simulink model "Dinamic_3_day_data_General"  (R2014b)
settings: Solver=ode45  StartTime=0.0  StopTime=255600  FixedStep=3600  RelTol=1e-3
undefined symbols (not defined in the file or in its folder): date_3, Dry_bulb_3, GHI_3
libraries: simulink x1
settings Model: Creator=Timur  LastModifiedBy=Timur
settings SolverCC: InitialStep=1000  ZeroCrossAlgorithm=Adaptive
settings DebuggingCC: AlgebraicLoopMsg=none  MaxConsecutiveZCsMsg=none  SolverPrmCheckMsg=none

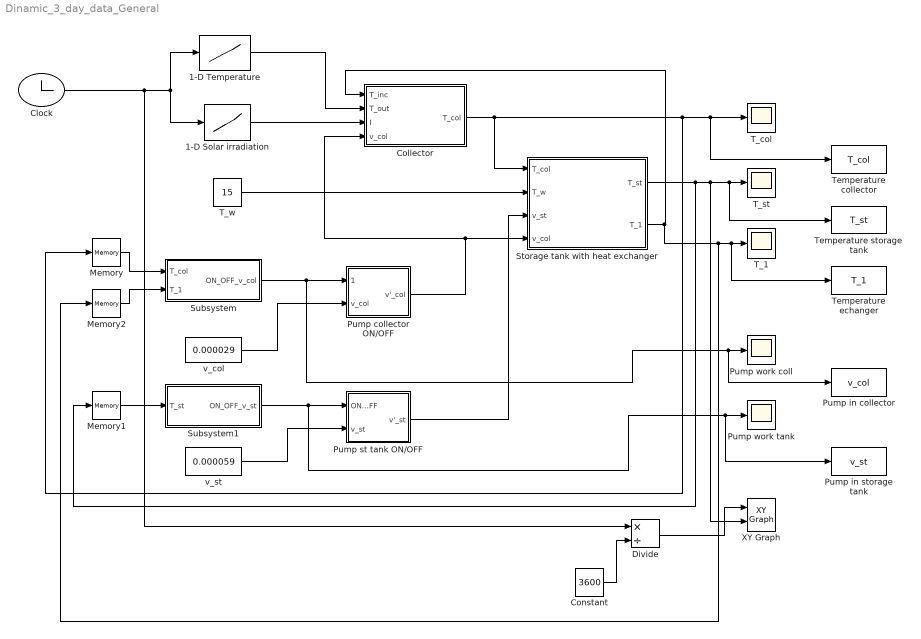
== system Dinamic_3_day_data_General ==
  1-D Solar irradiation : Lookup_n-D  NumberOfTableDimensions=1  BreakpointsForDimension1=date_3  Table=GHI_3  InterpMethod=Cubic spline  SampleTime=3600  InternalRulePriority=Speed  RndMeth=Simplest  InputSameDT=on
  1-D Temperature : Lookup_n-D  NumberOfTableDimensions=1  BreakpointsForDimension1=date_3  Table=Dry_bulb_3  InterpMethod=Cubic spline  SampleTime=3600  InternalRulePriority=Speed  RndMeth=Simplest  InputSameDT=on
  Clock : Clock
  Collector : Subsystem
  Constant : Constant  Value=3600
  Divide : Product  Inputs=*/
  Memory : Memory
  Memory1 : Memory
  Memory2 : Memory
  Pump collector ON/OFF : Subsystem
  Pump in collector : ToWorkspace  VariableName=v_col  SaveFormat=Timeseries  SampleTime=-1
  Pump in storage tank : ToWorkspace  VariableName=v_st  SaveFormat=Timeseries  SampleTime=-1
  Pump st tank ON/OFF : Subsystem
  Pump work coll : Scope
      settings: YMin=0  YMax=1  SaveName=ScopeData3
  Pump work tank : Scope
      settings: YMin=-1  YMax=1  SaveName=ScopeData4
  Storage tank with heat exchanger : Subsystem
  Subsystem : Subsystem
  Subsystem1 : Subsystem
  T_1 : Scope
      settings: YMin=10  YMax=60  SaveName=ScopeData2
  T_col : Scope
      settings: YMin=-80  YMax=100
  T_st : Scope
      settings: TimeRange=24  YMin=26.1999  YMax=26.2004
  T_w : Constant  Value=15
  Temperature collector : ToWorkspace  VariableName=T_col  SaveFormat=Timeseries  SampleTime=-1
  Temperature echanger : ToWorkspace  VariableName=T_1  SaveFormat=Timeseries  SampleTime=-1
  Temperature storage tank : ToWorkspace  VariableName=T_st  SaveFormat=Timeseries  SampleTime=-1
  XY Graph : simulink/Sinks/XY Graph  xmin=0  xmax=71  ymin=0  ymax=70  st=3600
  v_col : Constant  Value=0.000029
  v_st : Constant  Value=0.000059
  wires:
  1-D Temperature/1 -> Collector/2(T_out)
  v_col/1 -> Pump collector ON/OFF/2(v_col)
  Collector/1(T_col) -> Memory/1, Temperature collector/1, T_col/1, Storage tank with heat exchanger/1(T_col)
  T_w/1 -> Storage tank with heat exchanger/2(T_w)
  v_st/1 -> Pump st tank ON/OFF/2(v_st)
  Storage tank with heat exchanger/1(T_st) -> Memory1/1, XY Graph/2, Temperature storage tank/1, T_st/1
  Storage tank with heat exchanger/2(T_1) -> Memory2/1, Temperature echanger/1, T_1/1, Collector/1(T_inc)
  Pump collector ON/OFF/1(v'_col) -> Storage tank with heat exchanger/4(v_col), Collector/4(v_col)
  Subsystem/1(ON_OFF_v_col) -> Pump in collector/1, Pump work coll/1, Pump collector ON/OFF/1(ON_OFF)
  Pump st tank ON/OFF/1(v'_st) -> Storage tank with heat exchanger/3(v_st)
  Clock/1 -> 1-D Solar irradiation/1, 1-D Temperature/1, Divide/1
  1-D Solar irradiation/1 -> Collector/3(I)
  Constant/1 -> Divide/2
  Divide/1 -> XY Graph/1
  Subsystem1/1(ON_OFF_v_st) -> Pump work tank/1, Pump in storage tank/1, Pump st tank ON/OFF/1(ON_OFF)
  Memory/1 -> Subsystem/1(T_col)
  Memory1/1 -> Subsystem1/1(T_st)
  Memory2/1 -> Subsystem/2(T_1)

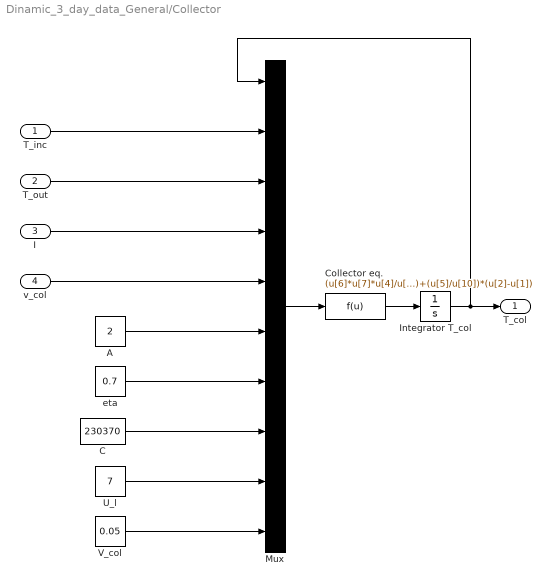
== system Dinamic_3_day_data_General/Collector ==
  T_inc : Inport
  T_out : Inport  Port=2
  I : Inport  Port=3
  v_col : Inport  Port=4
  A : Constant  Value=2
  C : Constant  Value=230370
  Collector eq. : Fcn  Expr=(u[6]*u[7]*u[4]/u[8])-((u[9]*u[6])/u[8])*((u[2]+u[1])/2-u[3])+(u[5]/u[10])*(u[2]-u[1])
  Integrator T_col : Integrator
  Mux : Mux  Inputs=10
  U_l : Constant  Value=7
  V_col : Constant  Value=0.05
  eta : Constant  Value=0.7
  T_col : Outport
  wires:
  T_inc/1 -> Mux/2
  T_out/1 -> Mux/3
  I/1 -> Mux/4
  v_col/1 -> Mux/5
  Mux/1 -> Collector eq./1
  Collector eq./1 -> Integrator T_col/1
  Integrator T_col/1 -> T_col/1, Mux/1
  A/1 -> Mux/6
  eta/1 -> Mux/7
  C/1 -> Mux/8
  U_l/1 -> Mux/9
  V_col/1 -> Mux/10

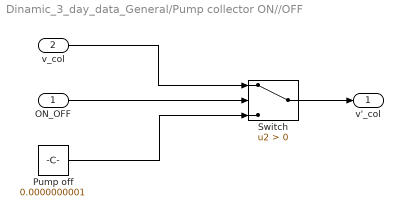
== system Dinamic_3_day_data_General/Pump collector ON//OFF ==
  ON_OFF : Inport
  v_col : Inport  Port=2
  Pump off : Constant  Value=0.0000000001
  Switch : Switch  Criteria=u2 > Threshold
  v'_col : Outport  OutMin=[0]
  wires:
  ON_OFF/1 -> Switch/2
  Pump off/1 -> Switch/3
  Switch/1 -> v'_col/1
  v_col/1 -> Switch/1

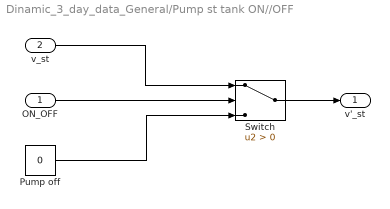
== system Dinamic_3_day_data_General/Pump st tank ON//OFF ==
  ON_OFF : Inport
  v_st : Inport  Port=2
  Pump off : Constant  Value=0
  Switch : Switch  Criteria=u2 > Threshold
  v'_st : Outport  OutMin=[0]
  wires:
  ON_OFF/1 -> Switch/2
  Pump off/1 -> Switch/3
  Switch/1 -> v'_st/1
  v_st/1 -> Switch/1

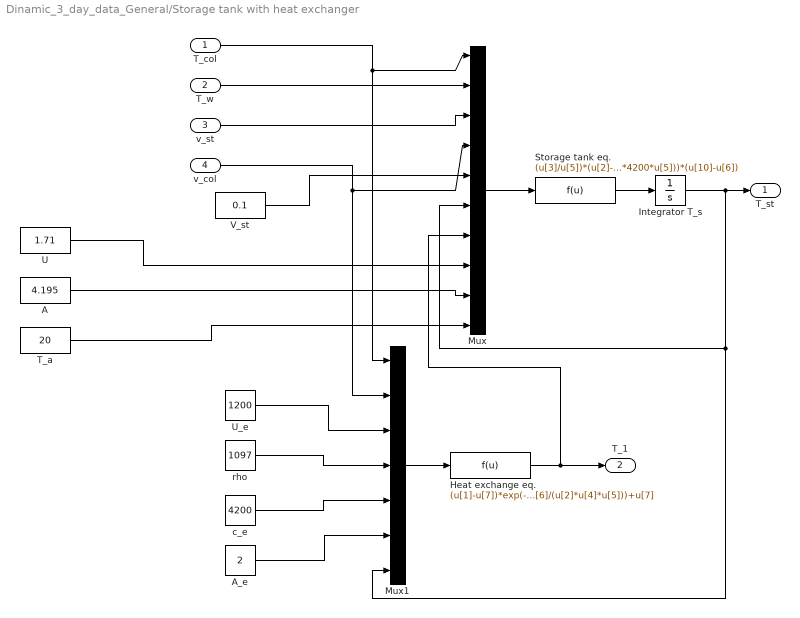
== system Dinamic_3_day_data_General/Storage tank with heat exchanger ==
  T_col : Inport
  T_w : Inport  Port=2
  v_st : Inport  Port=3
  v_col : Inport  Port=4
  A : Constant  Value=4.195
  A_e : Constant  Value=2
  Heat exchange eq. : Fcn  Expr=(u[1]-u[7])*exp(-u[3]*u[6]/(u[2]*u[4]*u[5]))+u[7]
  Integrator T_s : Integrator  InitialCondition=15  ZeroCross=off
  Mux : Mux  Inputs=10
  Mux1 : Mux  Inputs=7
  Storage tank eq. : Fcn  Expr=(u[3]/u[5])*(u[2]-u[6])+(u[4]/u[5])*(u[1]-u[7])+((u[8]*u[9])/(1097*4200*u[5]))*(u[10]-u[6])
  T_a : Constant  Value=20
  U : Constant  Value=1.71
  U_e : Constant  Value=1200
  V_st : Constant  Value=0.1
  c_e : Constant  Value=4200
  rho : Constant  Value=1097
  T_st : Outport  OutMin=[0]
  T_1 : Outport  Port=2  OutMin=[0]
  wires:
  T_col/1 -> Mux1/1, Mux/1
  T_w/1 -> Mux/2
  Mux/1 -> Storage tank eq./1
  v_st/1 -> Mux/3
  v_col/1 -> Mux1/2, Mux/4
  V_st/1 -> Mux/5
  U_e/1 -> Mux1/3
  rho/1 -> Mux1/4
  c_e/1 -> Mux1/5
  A_e/1 -> Mux1/6
  Mux1/1 -> Heat exchange eq./1
  Storage tank eq./1 -> Integrator T_s/1
  Heat exchange eq./1 -> Mux/7, T_1/1
  Integrator T_s/1 -> Mux1/7, Mux/6, T_st/1
  U/1 -> Mux/8
  A/1 -> Mux/9
  T_a/1 -> Mux/10

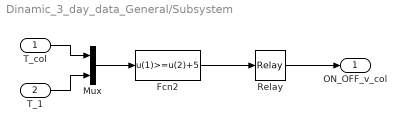
== system Dinamic_3_day_data_General/Subsystem ==
  T_col : Inport
  T_1 : Inport  Port=2
  Fcn2 : Fcn  Expr=u(1)>=u(2)+5
  Mux : Mux  Inputs=2
  Relay : Relay  OnSwitchValue=1  OffSwitchValue=0
  ON_OFF_v_col : Outport
  wires:
  T_col/1 -> Mux/1
  Relay/1 -> ON_OFF_v_col/1
  Fcn2/1 -> Relay/1
  T_1/1 -> Mux/2
  Mux/1 -> Fcn2/1

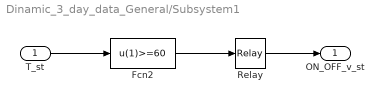
== system Dinamic_3_day_data_General/Subsystem1 ==
  T_st : Inport
  Fcn2 : Fcn  Expr=u(1)>=60
  Relay : Relay  OnSwitchValue=1  OffSwitchValue=0
  ON_OFF_v_st : Outport
  wires:
  T_st/1 -> Fcn2/1
  Fcn2/1 -> Relay/1
  Relay/1 -> ON_OFF_v_st/1
